simulink model "DY05S600_robot_controller_main_opensource"  (R2020a)
settings: Solver=FixedStepAuto  StartTime=0.0  StopTime=inf  FixedStep=SAMPLE_TIME  RelTol=1e-3
(part 2 of 2)

== matlab function DY05S600_robot_controller_main_opensource/ATS_controller/fuzzy_membership_function12 ==
  data: x input; beta output; wdot output
function [beta,wdot] = fcn(x)

%xm是规则中心
xm=zeros(5,4);
for j=1:5
    xm(j,1)=-0.26+0.13*(j-1)+0.1;
end
for j=6:10
    xm(j-5,2)=-0.18+0.09*(j-5-1)+0.1;
end
for j=11:15
    xm(j-10,3)=-0.14+0.07*(j-10-1)+0.1;
end
for j=16:20
    xm(j-15,4)=-0.4+0.2*(j-15-1)+0.1;
end



%xm是规则中心从小值到大值排列,x是前件变量,
r=length(xm(:,1)); %length(xm)是规则数量r
n=length(xm(1,:));%length(x)是前件变量维度
%初始化隶属度函数
ux=zeros(r,n);

for k=1:n
    if x(k)<=xm(1,k)   %论域左边界外
        ux(1,k)=1;
    end
    if x(k)>=xm(r,k)   %论域右边界外
        ux(r,k)=1;
    end
    for i=1:r-1  %从左到右只计算下降的隶属度函数
        if x(k)>=xm(i,k)&&x(k)<=xm(i+1,k)
           ux(i,k)=0.5*sin(pi*(x(k)-xm(i,k))/abs(xm(i,k)-xm(i+1,k))+0.5*pi)+0.5; %一种具有一阶可导性的四边形家族隶属度函数
        end
    end
    for i=2:r  %从左到右只计算上升的隶属度函数
        if x(k)>=xm(i-1,k)&&x(k)<=xm(i,k)
           ux(i,k)=0.5*sin(pi*(x(k)-xm(i,k))/abs(xm(i-1,k)-xm(i,k))+0.5*pi)+0.5;
        end
    end
end

kx=1;
jz=1;
[beta,wdot]= fuzzyoutput(ux,x,xm,kx,jz);

% function  [Basic,beta]= sumfuzzy_test(x) 
% ux=x;
% im=1;
% jm=0;
% bias=1;
% Basic=0;
% dem=length(ux(:,1))^length(ux(1,:)); %隶属度函数的重数数量
% beta=zeros(dem,1);
% [Basic,beta] = myfun(im,jm,ux,bias,Basic,beta);
% function [Basic,beta,jm] = myfun(im,jm,ux,bias,Basic,beta) 
% %针对ux隶属度函数矩阵的中心平均解模糊，初值赋为1,0，ux，1，0，执行的是多重求和
%     if  im > length(ux(1,:))    %length(ux(1,:))为前件输入的维度
%         Basic = Basic + bias;
%         jm=jm+1;                %相对于i1...in规则编号，此处是从最后一列填满到第一列（i1,...,in）
%         beta(jm,1)=bias;        %beta(i1,...,in)*xk*z(i6,j)
%     else
%         for km=1:length(ux(:,1))   %length(ux(:,1))为规则数量
%             bias_last = bias;
%             bias = bias* ux(km,im);
%             im = im+1;
%             [Basic,beta,jm] = myfun(im,jm,ux,bias,Basic,beta); %递归，拦在这里一直到function执行结束,每执行一次就会多一个for循环（每次跳出就是再一次的for内循环）
%             im = im-1; 
%             bias  = bias_last;
%         end
%     end
% end


end

== matlab function DY05S600_robot_controller_main_opensource/ATS_controller/fuzzy_membership_function9 ==
  data: x input; beta output; wdot output
function [beta,wdot] = fcn(x)

%xm是规则中心
xm=zeros(5,4);
for j=1:5
    xm(j,1)=-0.26+0.13*(j-1)+0.1;
end
for j=6:10
    xm(j-5,2)=-0.18+0.09*(j-5-1)+0.1;
end
for j=11:15
    xm(j-10,3)=-0.14+0.07*(j-10-1)+0.1;
end
for j=16:20
    xm(j-15,4)=-0.4+0.2*(j-15-1)+0.1;
end



%xm是规则中心从小值到大值排列,x是前件变量,
r=length(xm(:,1)); %length(xm)是规则数量r
n=length(xm(1,:));%length(x)是前件变量维度
%初始化隶属度函数
ux=zeros(r,n);

for k=1:n
    if x(k)<=xm(1,k)   %论域左边界外
        ux(1,k)=1;
    end
    if x(k)>=xm(r,k)   %论域右边界外
        ux(r,k)=1;
    end
    for i=1:r-1  %从左到右只计算下降的隶属度函数
        if x(k)>=xm(i,k)&&x(k)<=xm(i+1,k)
           ux(i,k)=0.5*sin(pi*(x(k)-xm(i,k))/abs(xm(i,k)-xm(i+1,k))+0.5*pi)+0.5; %一种具有一阶可导性的四边形家族隶属度函数
        end
    end
    for i=2:r  %从左到右只计算上升的隶属度函数
        if x(k)>=xm(i-1,k)&&x(k)<=xm(i,k)
           ux(i,k)=0.5*sin(pi*(x(k)-xm(i,k))/abs(xm(i-1,k)-xm(i,k))+0.5*pi)+0.5;
        end
    end
end

kx=1;
jz=1;
[beta,wdot]= fuzzyoutput(ux,x,xm,kx,jz);

% function  [Basic,beta]= sumfuzzy_test(x) 
% ux=x;
% im=1;
% jm=0;
% bias=1;
% Basic=0;
% dem=length(ux(:,1))^length(ux(1,:)); %隶属度函数的重数数量
% beta=zeros(dem,1);
% [Basic,beta] = myfun(im,jm,ux,bias,Basic,beta);
% function [Basic,beta,jm] = myfun(im,jm,ux,bias,Basic,beta) 
% %针对ux隶属度函数矩阵的中心平均解模糊，初值赋为1,0，ux，1，0，执行的是多重求和
%     if  im > length(ux(1,:))    %length(ux(1,:))为前件输入的维度
%         Basic = Basic + bias;
%         jm=jm+1;                %相对于i1...in规则编号，此处是从最后一列填满到第一列（i1,...,in）
%         beta(jm,1)=bias;        %beta(i1,...,in)*xk*z(i6,j)
%     else
%         for km=1:length(ux(:,1))   %length(ux(:,1))为规则数量
%             bias_last = bias;
%             bias = bias* ux(km,im);
%             im = im+1;
%             [Basic,beta,jm] = myfun(im,jm,ux,bias,Basic,beta); %递归，拦在这里一直到function执行结束,每执行一次就会多一个for循环（每次跳出就是再一次的for内循环）
%             im = im-1; 
%             bias  = bias_last;
%         end
%     end
% end


end

== matlab function DY05S600_robot_controller_main_opensource/ATS_controller/TSfuzzy_system_output13 ==
  data: beta input; w input; AF11 output
function AF11  = fcn(beta,w)

AF11=0;
for i=1:length(beta)
    AF11=AF11+w(i,1)*beta(i,1);
end

end

== matlab function DY05S600_robot_controller_main_opensource/ATS_controller/TSfuzzy_system_output14 ==
  data: beta input; w input; AF11 output
function AF11  = fcn(beta,w)

AF11=0;
for i=1:length(beta)
    AF11=AF11+w(i,1)*beta(i,1);
end

end

== matlab function DY05S600_robot_controller_main_opensource/ATS_controller/TSfuzzy_system_output15 ==
  data: beta input; w input; AF11 output
function AF11  = fcn(beta,w)

AF11=0;
for i=1:length(beta)
    AF11=AF11+w(i,1)*beta(i,1);
end

end

== matlab function DY05S600_robot_controller_main_opensource/ATS_controller/TSfuzzy_system_output16 ==
  data: beta input; w input; AF11 output
function AF11  = fcn(beta,w)

AF11=0;
for i=1:length(beta)
    AF11=AF11+w(i,1)*beta(i,1);
end

end

== matlab function DY05S600_robot_controller_main_opensource/ATS_controller/controller4 ==
  data: AF11 input; AF12 input; AF21 input; AF22 input; K1 input; K2 input; u1 output; u2 output; x1 input; x2 input; dag output
function [u1,u2,dag]  = fcn(AF11,AF12,AF21,AF22,K1,K2,x1,x2)

b1=0.1;
b2=0.01;

dag=0.8*pi/180;

% u1=-1/b1*((0+AF11)*x1+(0+AF12)*x2+K1*x1/dag^2);
% 
% u2=-1/b2*((0+AF21)*x1+(0+AF22)*x2+K2*x2/dag^2);

% dagx1=0.5*pi/180;
% satx1=0;
% if abs(x1)<dagx1
%     satx1=sign(x1);
% else
%     satx1=x1/dagx1;
% end

   
u1=-1/b1*((0.3+AF11)*x1+(0+AF12)*x2+K1*4/pi*atan(x1/dag));

u2=-1/b2*((2+AF21)*x1+(0.4+AF22)*x2+K2*4/pi*atan(x2/dag));


end

== matlab function DY05S600_robot_controller_main_opensource/ATS_controller/fuzzy_membership_function13 ==
  data: x input; beta output; wdot output
function [beta,wdot] = fcn(x)

%xm是规则中心
xm=zeros(5,4);
for j=1:5
    xm(j,1)=-0.26+0.13*(j-1)+0.1;
end
for j=6:10
    xm(j-5,2)=-0.18+0.09*(j-5-1)+0.1;
end
for j=11:15
    xm(j-10,3)=-0.14+0.07*(j-10-1)+0.1;
end
for j=16:20
    xm(j-15,4)=-0.4+0.2*(j-15-1)+0.1;
end



%xm是规则中心从小值到大值排列,x是前件变量,
r=length(xm(:,1)); %length(xm)是规则数量r
n=length(xm(1,:));%length(x)是前件变量维度
%初始化隶属度函数
ux=zeros(r,n);

for k=1:n
    if x(k)<=xm(1,k)   %论域左边界外
        ux(1,k)=1;
    end
    if x(k)>=xm(r,k)   %论域右边界外
        ux(r,k)=1;
    end
    for i=1:r-1  %从左到右只计算下降的隶属度函数
        if x(k)>=xm(i,k)&&x(k)<=xm(i+1,k)
           ux(i,k)=0.5*sin(pi*(x(k)-xm(i,k))/abs(xm(i,k)-xm(i+1,k))+0.5*pi)+0.5; %一种具有一阶可导性的四边形家族隶属度函数
        end
    end
    for i=2:r  %从左到右只计算上升的隶属度函数
        if x(k)>=xm(i-1,k)&&x(k)<=xm(i,k)
           ux(i,k)=0.5*sin(pi*(x(k)-xm(i,k))/abs(xm(i-1,k)-xm(i,k))+0.5*pi)+0.5;
        end
    end
end

kx=1;
jz=1;
[beta,wdot]= fuzzyoutput(ux,x,xm,kx,jz);

% function  [Basic,beta]= sumfuzzy_test(x) 
% ux=x;
% im=1;
% jm=0;
% bias=1;
% Basic=0;
% dem=length(ux(:,1))^length(ux(1,:)); %隶属度函数的重数数量
% beta=zeros(dem,1);
% [Basic,beta] = myfun(im,jm,ux,bias,Basic,beta);
% function [Basic,beta,jm] = myfun(im,jm,ux,bias,Basic,beta) 
% %针对ux隶属度函数矩阵的中心平均解模糊，初值赋为1,0，ux，1，0，执行的是多重求和
%     if  im > length(ux(1,:))    %length(ux(1,:))为前件输入的维度
%         Basic = Basic + bias;
%         jm=jm+1;                %相对于i1...in规则编号，此处是从最后一列填满到第一列（i1,...,in）
%         beta(jm,1)=bias;        %beta(i1,...,in)*xk*z(i6,j)
%     else
%         for km=1:length(ux(:,1))   %length(ux(:,1))为规则数量
%             bias_last = bias;
%             bias = bias* ux(km,im);
%             im = im+1;
%             [Basic,beta,jm] = myfun(im,jm,ux,bias,Basic,beta); %递归，拦在这里一直到function执行结束,每执行一次就会多一个for循环（每次跳出就是再一次的for内循环）
%             im = im-1; 
%             bias  = bias_last;
%         end
%     end
% end


end

== matlab function DY05S600_robot_controller_main_opensource/ATS_controller/fuzzy_membership_function14 ==
  data: x input; beta output; wdot output
function [beta,wdot] = fcn(x)

%xm是规则中心
xm=zeros(5,4);
for j=1:5
    xm(j,1)=-0.26+0.13*(j-1)+0.1;
end
for j=6:10
    xm(j-5,2)=-0.18+0.09*(j-5-1)+0.1;
end
for j=11:15
    xm(j-10,3)=-0.14+0.07*(j-10-1)+0.1;
end
for j=16:20
    xm(j-15,4)=-0.4+0.2*(j-15-1)+0.1;
end



%xm是规则中心从小值到大值排列,x是前件变量,
r=length(xm(:,1)); %length(xm)是规则数量r
n=length(xm(1,:));%length(x)是前件变量维度
%初始化隶属度函数
ux=zeros(r,n);

for k=1:n
    if x(k)<=xm(1,k)   %论域左边界外
        ux(1,k)=1;
    end
    if x(k)>=xm(r,k)   %论域右边界外
        ux(r,k)=1;
    end
    for i=1:r-1  %从左到右只计算下降的隶属度函数
        if x(k)>=xm(i,k)&&x(k)<=xm(i+1,k)
           ux(i,k)=0.5*sin(pi*(x(k)-xm(i,k))/abs(xm(i,k)-xm(i+1,k))+0.5*pi)+0.5; %一种具有一阶可导性的四边形家族隶属度函数
        end
    end
    for i=2:r  %从左到右只计算上升的隶属度函数
        if x(k)>=xm(i-1,k)&&x(k)<=xm(i,k)
           ux(i,k)=0.5*sin(pi*(x(k)-xm(i,k))/abs(xm(i-1,k)-xm(i,k))+0.5*pi)+0.5;
        end
    end
end

kx=1;
jz=1;
[beta,wdot]= fuzzyoutput(ux,x,xm,kx,jz);

% function  [Basic,beta]= sumfuzzy_test(x) 
% ux=x;
% im=1;
% jm=0;
% bias=1;
% Basic=0;
% dem=length(ux(:,1))^length(ux(1,:)); %隶属度函数的重数数量
% beta=zeros(dem,1);
% [Basic,beta] = myfun(im,jm,ux,bias,Basic,beta);
% function [Basic,beta,jm] = myfun(im,jm,ux,bias,Basic,beta) 
% %针对ux隶属度函数矩阵的中心平均解模糊，初值赋为1,0，ux，1，0，执行的是多重求和
%     if  im > length(ux(1,:))    %length(ux(1,:))为前件输入的维度
%         Basic = Basic + bias;
%         jm=jm+1;                %相对于i1...in规则编号，此处是从最后一列填满到第一列（i1,...,in）
%         beta(jm,1)=bias;        %beta(i1,...,in)*xk*z(i6,j)
%     else
%         for km=1:length(ux(:,1))   %length(ux(:,1))为规则数量
%             bias_last = bias;
%             bias = bias* ux(km,im);
%             im = im+1;
%             [Basic,beta,jm] = myfun(im,jm,ux,bias,Basic,beta); %递归，拦在这里一直到function执行结束,每执行一次就会多一个for循环（每次跳出就是再一次的for内循环）
%             im = im-1; 
%             bias  = bias_last;
%         end
%     end
% end


end

== matlab function DY05S600_robot_controller_main_opensource/ATS_controller/fuzzy_membership_function15 ==
  data: x input; beta output; wdot output
function [beta,wdot] = fcn(x)

%xm是规则中心
xm=zeros(5,4);
for j=1:5
    xm(j,1)=-0.26+0.13*(j-1)+0.1;
end
for j=6:10
    xm(j-5,2)=-0.18+0.09*(j-5-1)+0.1;
end
for j=11:15
    xm(j-10,3)=-0.14+0.07*(j-10-1)+0.1;
end
for j=16:20
    xm(j-15,4)=-0.4+0.2*(j-15-1)+0.1;
end


%xm是规则中心从小值到大值排列,x是前件变量,
r=length(xm(:,1)); %length(xm)是规则数量r
n=length(xm(1,:));%length(x)是前件变量维度
%初始化隶属度函数
ux=zeros(r,n);

for k=1:n
    if x(k)<=xm(1,k)   %论域左边界外
        ux(1,k)=1;
    end
    if x(k)>=xm(r,k)   %论域右边界外
        ux(r,k)=1;
    end
    for i=1:r-1  %从左到右只计算下降的隶属度函数
        if x(k)>=xm(i,k)&&x(k)<=xm(i+1,k)
           ux(i,k)=0.5*sin(pi*(x(k)-xm(i,k))/abs(xm(i,k)-xm(i+1,k))+0.5*pi)+0.5; %一种具有一阶可导性的四边形家族隶属度函数
        end
    end
    for i=2:r  %从左到右只计算上升的隶属度函数
        if x(k)>=xm(i-1,k)&&x(k)<=xm(i,k)
           ux(i,k)=0.5*sin(pi*(x(k)-xm(i,k))/abs(xm(i-1,k)-xm(i,k))+0.5*pi)+0.5;
        end
    end
end

kx=1;
jz=1;
[beta,wdot]= fuzzyoutput(ux,x,xm,kx,jz);

% function  [Basic,beta]= sumfuzzy_test(x) 
% ux=x;
% im=1;
% jm=0;
% bias=1;
% Basic=0;
% dem=length(ux(:,1))^length(ux(1,:)); %隶属度函数的重数数量
% beta=zeros(dem,1);
% [Basic,beta] = myfun(im,jm,ux,bias,Basic,beta);
% function [Basic,beta,jm] = myfun(im,jm,ux,bias,Basic,beta) 
% %针对ux隶属度函数矩阵的中心平均解模糊，初值赋为1,0，ux，1，0，执行的是多重求和
%     if  im > length(ux(1,:))    %length(ux(1,:))为前件输入的维度
%         Basic = Basic + bias;
%         jm=jm+1;                %相对于i1...in规则编号，此处是从最后一列填满到第一列（i1,...,in）
%         beta(jm,1)=bias;        %beta(i1,...,in)*xk*z(i6,j)
%     else
%         for km=1:length(ux(:,1))   %length(ux(:,1))为规则数量
%             bias_last = bias;
%             bias = bias* ux(km,im);
%             im = im+1;
%             [Basic,beta,jm] = myfun(im,jm,ux,bias,Basic,beta); %递归，拦在这里一直到function执行结束,每执行一次就会多一个for循环（每次跳出就是再一次的for内循环）
%             im = im-1; 
%             bias  = bias_last;
%         end
%     end
% end


end

== matlab function DY05S600_robot_controller_main_opensource/ATS_controller/fuzzy_membership_function16 ==
  data: x input; beta output; wdot output
function [beta,wdot] = fcn(x)

%xm是规则中心
xm=zeros(5,4);
for j=1:5
    xm(j,1)=-0.26+0.13*(j-1)+0.1;
end
for j=6:10
    xm(j-5,2)=-0.18+0.09*(j-5-1)+0.1;
end
for j=11:15
    xm(j-10,3)=-0.14+0.07*(j-10-1)+0.1;
end
for j=16:20
    xm(j-15,4)=-0.4+0.2*(j-15-1)+0.1;
end



%xm是规则中心从小值到大值排列,x是前件变量,
r=length(xm(:,1)); %length(xm)是规则数量r
n=length(xm(1,:));%length(x)是前件变量维度
%初始化隶属度函数
ux=zeros(r,n);

for k=1:n
    if x(k)<=xm(1,k)   %论域左边界外
        ux(1,k)=1;
    end
    if x(k)>=xm(r,k)   %论域右边界外
        ux(r,k)=1;
    end
    for i=1:r-1  %从左到右只计算下降的隶属度函数
        if x(k)>=xm(i,k)&&x(k)<=xm(i+1,k)
           ux(i,k)=0.5*sin(pi*(x(k)-xm(i,k))/abs(xm(i,k)-xm(i+1,k))+0.5*pi)+0.5; %一种具有一阶可导性的四边形家族隶属度函数
        end
    end
    for i=2:r  %从左到右只计算上升的隶属度函数
        if x(k)>=xm(i-1,k)&&x(k)<=xm(i,k)
           ux(i,k)=0.5*sin(pi*(x(k)-xm(i,k))/abs(xm(i-1,k)-xm(i,k))+0.5*pi)+0.5;
        end
    end
end

kx=1;
jz=1;
[beta,wdot]= fuzzyoutput(ux,x,xm,kx,jz);

% function  [Basic,beta]= sumfuzzy_test(x) 
% ux=x;
% im=1;
% jm=0;
% bias=1;
% Basic=0;
% dem=length(ux(:,1))^length(ux(1,:)); %隶属度函数的重数数量
% beta=zeros(dem,1);
% [Basic,beta] = myfun(im,jm,ux,bias,Basic,beta);
% function [Basic,beta,jm] = myfun(im,jm,ux,bias,Basic,beta) 
% %针对ux隶属度函数矩阵的中心平均解模糊，初值赋为1,0，ux，1，0，执行的是多重求和
%     if  im > length(ux(1,:))    %length(ux(1,:))为前件输入的维度
%         Basic = Basic + bias;
%         jm=jm+1;                %相对于i1...in规则编号，此处是从最后一列填满到第一列（i1,...,in）
%         beta(jm,1)=bias;        %beta(i1,...,in)*xk*z(i6,j)
%     else
%         for km=1:length(ux(:,1))   %length(ux(:,1))为规则数量
%             bias_last = bias;
%             bias = bias* ux(km,im);
%             im = im+1;
%             [Basic,beta,jm] = myfun(im,jm,ux,bias,Basic,beta); %递归，拦在这里一直到function执行结束,每执行一次就会多一个for循环（每次跳出就是再一次的for内循环）
%             im = im-1; 
%             bias  = bias_last;
%         end
%     end
% end


end

== matlab function DY05S600_robot_controller_main_opensource/ATS_controller/K_comp1 ==
  data: k1 input; x1 input; x2 input; y output; k2 input
function y   = fcn(k1,x1,x2,k2)

x=abs(x1*180/pi)-0.01;

ux=zeros(13,1);
%%x1 13条模糊规则
h1=0.2;%%规则间距


if x<=0
    ux(1,1)=1;
end

if x>=0&&x<=0.2
    ux(1,1)=0.5*sin(pi*(x-(0))/h1+0.5*pi)+0.5;
end

if x>=0&&x<=0.4
    ux(2,1)=0.5*sin(pi*(x-(0.2))/h1+0.5*pi)+0.5;
end

if x>=0.2&&x<=0.6
    ux(3,1)=0.5*sin(pi*(x-(0.4))/h1+0.5*pi)+0.5;
end

if x>=0.4&&x<=0.8
    ux(4,1)=0.5*sin(pi*(x-(0.6))/h1+0.5*pi)+0.5;
end

if x>=0.6&&x<=1
    ux(5,1)=0.5*sin(pi*(x-(0.8))/h1+0.5*pi)+0.5;
end

if x>=0.8&&x<=1.2
    ux(6,1)=0.5*sin(pi*(x-(1))/h1+0.5*pi)+0.5;
end

if x>=1&&x<=1.4
    ux(7,1)=0.5*sin(pi*(x-(1.2))/h1+0.5*pi)+0.5;
end

if x>=1.2&&x<=1.6
    ux(8,1)=0.5*sin(pi*(x-(1.4))/h1+0.5*pi)+0.5;
end

if x>=1.4&&x<=1.8
    ux(9,1)=0.5*sin(pi*(x-(1.6))/h1+0.5*pi)+0.5;
end

if x>=1.6&&x<=2
    ux(10,1)=0.5*sin(pi*(x-(1.8))/h1+0.5*pi)+0.5;
end

if x>=1.8&&x<=2.2
    ux(11,1)=0.5*sin(pi*(x-(2))/h1+0.5*pi)+0.5;
end

if x>=2&&x<=2.4
    ux(12,1)=0.5*sin(pi*(x-(2.2))/h1+0.5*pi)+0.5;
end

if x>=2.2&&x<=2.4
    ux(13,1)=0.5*sin(pi*(x-(2.4))/h1+0.5*pi)+0.5;
end

if x>2.4
    ux(13,1)=1;
end

%中心平均解模糊
Basic=0;
for i=1:13
    Basic=Basic+ux(i,1);
end

beta=zeros(13,1);
for i=1:13
    beta(i,1)=ux(i,1)/Basic;
end

w=[0;1;0.95;0.9;0.85;0.8;0.75;0.7;0.65;0.6;0.55;0.5;0.45/exp(-2.4)*exp(-x)];

f=0;
for i=1:13
    f=f+w(i,1)*beta(i,1);
end

y1=f*k1;
y2=f*k2;
y=[y1,y2]';

end

== matlab function DY05S600_robot_controller_main_opensource/ATS_controller/TSfuzzy_system_output17 ==
  data: beta input; w input; AF11 output
function AF11  = fcn(beta,w)

AF11=0;
for i=1:length(beta)
    AF11=AF11+w(i,1)*beta(i,1);
end

end

== matlab function DY05S600_robot_controller_main_opensource/ATS_controller/TSfuzzy_system_output18 ==
  data: beta input; w input; AF11 output
function AF11  = fcn(beta,w)

AF11=0;
for i=1:length(beta)
    AF11=AF11+w(i,1)*beta(i,1);
end

end

== matlab function DY05S600_robot_controller_main_opensource/ATS_controller/TSfuzzy_system_output19 ==
  data: beta input; w input; AF11 output
function AF11  = fcn(beta,w)

AF11=0;
for i=1:length(beta)
    AF11=AF11+w(i,1)*beta(i,1);
end

end

== matlab function DY05S600_robot_controller_main_opensource/ATS_controller/TSfuzzy_system_output20 ==
  data: beta input; w input; AF11 output
function AF11  = fcn(beta,w)

AF11=0;
for i=1:length(beta)
    AF11=AF11+w(i,1)*beta(i,1);
end

end

== matlab function DY05S600_robot_controller_main_opensource/ATS_controller/controller5 ==
  data: AF11 input; AF12 input; AF21 input; AF22 input; K1 input; K2 input; u1 output; u2 output; x1 input; x2 input; dag output
function [u1,u2,dag]  = fcn(AF11,AF12,AF21,AF22,K1,K2,x1,x2)

b1=0.1;
b2=0.01;

dag=1*pi/180;

% u1=-1/b1*((0+AF11)*x1+(0+AF12)*x2+K1*x1/dag^2);
% 
% u2=-1/b2*((0+AF21)*x1+(0+AF22)*x2+K2*x2/dag^2);

% dagx1=0.5*pi/180;
% satx1=0;
% if abs(x1)<dagx1
%     satx1=sign(x1);
% else
%     satx1=x1/dagx1;
% end

   
u1=-1/b1*((0.1+AF11)*x1+(0+AF12)*x2+K1*4/pi*atan(x1/dag));

u2=-1/b2*((2+AF21)*x1+(0.1+AF22)*x2+K2*4/pi*atan(x2/dag));


end

== matlab function DY05S600_robot_controller_main_opensource/ATS_controller/fuzzy_membership_function17 ==
  data: x input; beta output; wdot output
function [beta,wdot] = fcn(x)

%xm是规则中心
xm=zeros(5,4);
for j=1:5
    xm(j,1)=-0.26+0.13*(j-1)+0.1;
end
for j=6:10
    xm(j-5,2)=-0.18+0.09*(j-5-1)+0.1;
end
for j=11:15
    xm(j-10,3)=-0.14+0.07*(j-10-1)+0.1;
end
for j=16:20
    xm(j-15,4)=-0.4+0.2*(j-15-1)+0.1;
end



%xm是规则中心从小值到大值排列,x是前件变量,
r=length(xm(:,1)); %length(xm)是规则数量r
n=length(xm(1,:));%length(x)是前件变量维度
%初始化隶属度函数
ux=zeros(r,n);

for k=1:n
    if x(k)<=xm(1,k)   %论域左边界外
        ux(1,k)=1;
    end
    if x(k)>=xm(r,k)   %论域右边界外
        ux(r,k)=1;
    end
    for i=1:r-1  %从左到右只计算下降的隶属度函数
        if x(k)>=xm(i,k)&&x(k)<=xm(i+1,k)
           ux(i,k)=0.5*sin(pi*(x(k)-xm(i,k))/abs(xm(i,k)-xm(i+1,k))+0.5*pi)+0.5; %一种具有一阶可导性的四边形家族隶属度函数
        end
    end
    for i=2:r  %从左到右只计算上升的隶属度函数
        if x(k)>=xm(i-1,k)&&x(k)<=xm(i,k)
           ux(i,k)=0.5*sin(pi*(x(k)-xm(i,k))/abs(xm(i-1,k)-xm(i,k))+0.5*pi)+0.5;
        end
    end
end

kx=1;
jz=1;
[beta,wdot]= fuzzyoutput(ux,x,xm,kx,jz);

% function  [Basic,beta]= sumfuzzy_test(x) 
% ux=x;
% im=1;
% jm=0;
% bias=1;
% Basic=0;
% dem=length(ux(:,1))^length(ux(1,:)); %隶属度函数的重数数量
% beta=zeros(dem,1);
% [Basic,beta] = myfun(im,jm,ux,bias,Basic,beta);
% function [Basic,beta,jm] = myfun(im,jm,ux,bias,Basic,beta) 
% %针对ux隶属度函数矩阵的中心平均解模糊，初值赋为1,0，ux，1，0，执行的是多重求和
%     if  im > length(ux(1,:))    %length(ux(1,:))为前件输入的维度
%         Basic = Basic + bias;
%         jm=jm+1;                %相对于i1...in规则编号，此处是从最后一列填满到第一列（i1,...,in）
%         beta(jm,1)=bias;        %beta(i1,...,in)*xk*z(i6,j)
%     else
%         for km=1:length(ux(:,1))   %length(ux(:,1))为规则数量
%             bias_last = bias;
%             bias = bias* ux(km,im);
%             im = im+1;
%             [Basic,beta,jm] = myfun(im,jm,ux,bias,Basic,beta); %递归，拦在这里一直到function执行结束,每执行一次就会多一个for循环（每次跳出就是再一次的for内循环）
%             im = im-1; 
%             bias  = bias_last;
%         end
%     end
% end


end

== matlab function DY05S600_robot_controller_main_opensource/ATS_controller/fuzzy_membership_function18 ==
  data: x input; beta output; wdot output
function [beta,wdot] = fcn(x)

%xm是规则中心
xm=zeros(5,4);
for j=1:5
    xm(j,1)=-0.26+0.13*(j-1)+0.1;
end
for j=6:10
    xm(j-5,2)=-0.18+0.09*(j-5-1)+0.1;
end
for j=11:15
    xm(j-10,3)=-0.14+0.07*(j-10-1)+0.1;
end
for j=16:20
    xm(j-15,4)=-0.4+0.2*(j-15-1)+0.1;
end



%xm是规则中心从小值到大值排列,x是前件变量,
r=length(xm(:,1)); %length(xm)是规则数量r
n=length(xm(1,:));%length(x)是前件变量维度
%初始化隶属度函数
ux=zeros(r,n);

for k=1:n
    if x(k)<=xm(1,k)   %论域左边界外
        ux(1,k)=1;
    end
    if x(k)>=xm(r,k)   %论域右边界外
        ux(r,k)=1;
    end
    for i=1:r-1  %从左到右只计算下降的隶属度函数
        if x(k)>=xm(i,k)&&x(k)<=xm(i+1,k)
           ux(i,k)=0.5*sin(pi*(x(k)-xm(i,k))/abs(xm(i,k)-xm(i+1,k))+0.5*pi)+0.5; %一种具有一阶可导性的四边形家族隶属度函数
        end
    end
    for i=2:r  %从左到右只计算上升的隶属度函数
        if x(k)>=xm(i-1,k)&&x(k)<=xm(i,k)
           ux(i,k)=0.5*sin(pi*(x(k)-xm(i,k))/abs(xm(i-1,k)-xm(i,k))+0.5*pi)+0.5;
        end
    end
end

kx=1;
jz=1;
[beta,wdot]= fuzzyoutput(ux,x,xm,kx,jz);

% function  [Basic,beta]= sumfuzzy_test(x) 
% ux=x;
% im=1;
% jm=0;
% bias=1;
% Basic=0;
% dem=length(ux(:,1))^length(ux(1,:)); %隶属度函数的重数数量
% beta=zeros(dem,1);
% [Basic,beta] = myfun(im,jm,ux,bias,Basic,beta);
% function [Basic,beta,jm] = myfun(im,jm,ux,bias,Basic,beta) 
% %针对ux隶属度函数矩阵的中心平均解模糊，初值赋为1,0，ux，1，0，执行的是多重求和
%     if  im > length(ux(1,:))    %length(ux(1,:))为前件输入的维度
%         Basic = Basic + bias;
%         jm=jm+1;                %相对于i1...in规则编号，此处是从最后一列填满到第一列（i1,...,in）
%         beta(jm,1)=bias;        %beta(i1,...,in)*xk*z(i6,j)
%     else
%         for km=1:length(ux(:,1))   %length(ux(:,1))为规则数量
%             bias_last = bias;
%             bias = bias* ux(km,im);
%             im = im+1;
%             [Basic,beta,jm] = myfun(im,jm,ux,bias,Basic,beta); %递归，拦在这里一直到function执行结束,每执行一次就会多一个for循环（每次跳出就是再一次的for内循环）
%             im = im-1; 
%             bias  = bias_last;
%         end
%     end
% end


end

== matlab function DY05S600_robot_controller_main_opensource/ATS_controller/fuzzy_membership_function19 ==
  data: x input; beta output; wdot output
function [beta,wdot] = fcn(x)

%xm是规则中心
xm=zeros(5,4);
for j=1:5
    xm(j,1)=-0.26+0.13*(j-1)+0.1;
end
for j=6:10
    xm(j-5,2)=-0.18+0.09*(j-5-1)+0.1;
end
for j=11:15
    xm(j-10,3)=-0.14+0.07*(j-10-1)+0.1;
end
for j=16:20
    xm(j-15,4)=-0.4+0.2*(j-15-1)+0.1;
end


%xm是规则中心从小值到大值排列,x是前件变量,
r=length(xm(:,1)); %length(xm)是规则数量r
n=length(xm(1,:));%length(x)是前件变量维度
%初始化隶属度函数
ux=zeros(r,n);

for k=1:n
    if x(k)<=xm(1,k)   %论域左边界外
        ux(1,k)=1;
    end
    if x(k)>=xm(r,k)   %论域右边界外
        ux(r,k)=1;
    end
    for i=1:r-1  %从左到右只计算下降的隶属度函数
        if x(k)>=xm(i,k)&&x(k)<=xm(i+1,k)
           ux(i,k)=0.5*sin(pi*(x(k)-xm(i,k))/abs(xm(i,k)-xm(i+1,k))+0.5*pi)+0.5; %一种具有一阶可导性的四边形家族隶属度函数
        end
    end
    for i=2:r  %从左到右只计算上升的隶属度函数
        if x(k)>=xm(i-1,k)&&x(k)<=xm(i,k)
           ux(i,k)=0.5*sin(pi*(x(k)-xm(i,k))/abs(xm(i-1,k)-xm(i,k))+0.5*pi)+0.5;
        end
    end
end

kx=1;
jz=1;
[beta,wdot]= fuzzyoutput(ux,x,xm,kx,jz);

% function  [Basic,beta]= sumfuzzy_test(x) 
% ux=x;
% im=1;
% jm=0;
% bias=1;
% Basic=0;
% dem=length(ux(:,1))^length(ux(1,:)); %隶属度函数的重数数量
% beta=zeros(dem,1);
% [Basic,beta] = myfun(im,jm,ux,bias,Basic,beta);
% function [Basic,beta,jm] = myfun(im,jm,ux,bias,Basic,beta) 
% %针对ux隶属度函数矩阵的中心平均解模糊，初值赋为1,0，ux，1，0，执行的是多重求和
%     if  im > length(ux(1,:))    %length(ux(1,:))为前件输入的维度
%         Basic = Basic + bias;
%         jm=jm+1;                %相对于i1...in规则编号，此处是从最后一列填满到第一列（i1,...,in）
%         beta(jm,1)=bias;        %beta(i1,...,in)*xk*z(i6,j)
%     else
%         for km=1:length(ux(:,1))   %length(ux(:,1))为规则数量
%             bias_last = bias;
%             bias = bias* ux(km,im);
%             im = im+1;
%             [Basic,beta,jm] = myfun(im,jm,ux,bias,Basic,beta); %递归，拦在这里一直到function执行结束,每执行一次就会多一个for循环（每次跳出就是再一次的for内循环）
%             im = im-1; 
%             bias  = bias_last;
%         end
%     end
% end


end

== matlab function DY05S600_robot_controller_main_opensource/ATS_controller/fuzzy_membership_function20 ==
  data: x input; beta output; wdot output
function [beta,wdot] = fcn(x)

%xm是规则中心
xm=zeros(5,4);
for j=1:5
    xm(j,1)=-0.26+0.13*(j-1)+0.1;
end
for j=6:10
    xm(j-5,2)=-0.18+0.09*(j-5-1)+0.1;
end
for j=11:15
    xm(j-10,3)=-0.14+0.07*(j-10-1)+0.1;
end
for j=16:20
    xm(j-15,4)=-0.4+0.2*(j-15-1)+0.1;
end



%xm是规则中心从小值到大值排列,x是前件变量,
r=length(xm(:,1)); %length(xm)是规则数量r
n=length(xm(1,:));%length(x)是前件变量维度
%初始化隶属度函数
ux=zeros(r,n);

for k=1:n
    if x(k)<=xm(1,k)   %论域左边界外
        ux(1,k)=1;
    end
    if x(k)>=xm(r,k)   %论域右边界外
        ux(r,k)=1;
    end
    for i=1:r-1  %从左到右只计算下降的隶属度函数
        if x(k)>=xm(i,k)&&x(k)<=xm(i+1,k)
           ux(i,k)=0.5*sin(pi*(x(k)-xm(i,k))/abs(xm(i,k)-xm(i+1,k))+0.5*pi)+0.5; %一种具有一阶可导性的四边形家族隶属度函数
        end
    end
    for i=2:r  %从左到右只计算上升的隶属度函数
        if x(k)>=xm(i-1,k)&&x(k)<=xm(i,k)
           ux(i,k)=0.5*sin(pi*(x(k)-xm(i,k))/abs(xm(i-1,k)-xm(i,k))+0.5*pi)+0.5;
        end
    end
end

kx=1;
jz=1;
[beta,wdot]= fuzzyoutput(ux,x,xm,kx,jz);

% function  [Basic,beta]= sumfuzzy_test(x) 
% ux=x;
% im=1;
% jm=0;
% bias=1;
% Basic=0;
% dem=length(ux(:,1))^length(ux(1,:)); %隶属度函数的重数数量
% beta=zeros(dem,1);
% [Basic,beta] = myfun(im,jm,ux,bias,Basic,beta);
% function [Basic,beta,jm] = myfun(im,jm,ux,bias,Basic,beta) 
% %针对ux隶属度函数矩阵的中心平均解模糊，初值赋为1,0，ux，1，0，执行的是多重求和
%     if  im > length(ux(1,:))    %length(ux(1,:))为前件输入的维度
%         Basic = Basic + bias;
%         jm=jm+1;                %相对于i1...in规则编号，此处是从最后一列填满到第一列（i1,...,in）
%         beta(jm,1)=bias;        %beta(i1,...,in)*xk*z(i6,j)
%     else
%         for km=1:length(ux(:,1))   %length(ux(:,1))为规则数量
%             bias_last = bias;
%             bias = bias* ux(km,im);
%             im = im+1;
%             [Basic,beta,jm] = myfun(im,jm,ux,bias,Basic,beta); %递归，拦在这里一直到function执行结束,每执行一次就会多一个for循环（每次跳出就是再一次的for内循环）
%             im = im-1; 
%             bias  = bias_last;
%         end
%     end
% end


end

== matlab function DY05S600_robot_controller_main_opensource/ATS_controller/TSfuzzy_system_output21 ==
  data: beta input; w input; AF11 output
function AF11  = fcn(beta,w)

AF11=0;
for i=1:length(beta)
    AF11=AF11+w(i,1)*beta(i,1);
end

end

== matlab function DY05S600_robot_controller_main_opensource/ATS_controller/TSfuzzy_system_output22 ==
  data: beta input; w input; AF11 output
function AF11  = fcn(beta,w)

AF11=0;
for i=1:length(beta)
    AF11=AF11+w(i,1)*beta(i,1);
end

end

== matlab function DY05S600_robot_controller_main_opensource/ATS_controller/TSfuzzy_system_output23 ==
  data: beta input; w input; AF11 output
function AF11  = fcn(beta,w)

AF11=0;
for i=1:length(beta)
    AF11=AF11+w(i,1)*beta(i,1);
end

end

== matlab function DY05S600_robot_controller_main_opensource/ATS_controller/TSfuzzy_system_output24 ==
  data: beta input; w input; AF11 output
function AF11  = fcn(beta,w)

AF11=0;
for i=1:length(beta)
    AF11=AF11+w(i,1)*beta(i,1);
end

end

== matlab function DY05S600_robot_controller_main_opensource/ATS_controller/controller6 ==
  data: AF11 input; AF12 input; AF21 input; AF22 input; K1 input; K2 input; u1 output; u2 output; x1 input; x2 input; dag output
function [u1,u2,dag]  = fcn(AF11,AF12,AF21,AF22,K1,K2,x1,x2)

b1=0.1;
b2=0.01;

dag=2.7*pi/180;

% u1=-1/b1*((0+AF11)*x1+(0+AF12)*x2+K1*x1/dag^2);
% 
% u2=-1/b2*((0+AF21)*x1+(0+AF22)*x2+K2*x2/dag^2);

% dagx1=0.5*pi/180;
% satx1=0;
% if abs(x1)<dagx1
%     satx1=sign(x1);
% else
%     satx1=x1/dagx1;
% end

% u1=-1/b1*((0.01+AF11)*x1+(0+AF12)*x2+K1*4/pi*atan(x1/dag));
% 
% 
% u2=-1/b2*((1+AF21)*x1+(0.01+AF22)*x2+K2*4/pi*atan(x2/dag));

u1=-1/b1*((0+0.1*AF11)*x1+(0+0.1*AF12)*x2+K1*4/pi*atan(x1/dag));


u2=-1/b2*((0.1+0.1*AF21)*x1+(0+0.1*AF22)*x2+K2*4/pi*atan(x2/dag));

end

== matlab function DY05S600_robot_controller_main_opensource/ATS_controller/fuzzy_membership_function21 ==
  data: x input; beta output; wdot output
function [beta,wdot] = fcn(x)

%xm是规则中心
xm=zeros(5,4);
for j=1:5
    xm(j,1)=-0.26+0.13*(j-1)+0.1;
end
for j=6:10
    xm(j-5,2)=-0.18+0.09*(j-5-1)+0.1;
end
for j=11:15
    xm(j-10,3)=-0.14+0.07*(j-10-1)+0.1;
end
for j=16:20
    xm(j-15,4)=-0.4+0.2*(j-15-1)+0.1;
end



%xm是规则中心从小值到大值排列,x是前件变量,
r=length(xm(:,1)); %length(xm)是规则数量r
n=length(xm(1,:));%length(x)是前件变量维度
%初始化隶属度函数
ux=zeros(r,n);

for k=1:n
    if x(k)<=xm(1,k)   %论域左边界外
        ux(1,k)=1;
    end
    if x(k)>=xm(r,k)   %论域右边界外
        ux(r,k)=1;
    end
    for i=1:r-1  %从左到右只计算下降的隶属度函数
        if x(k)>=xm(i,k)&&x(k)<=xm(i+1,k)
           ux(i,k)=0.5*sin(pi*(x(k)-xm(i,k))/abs(xm(i,k)-xm(i+1,k))+0.5*pi)+0.5; %一种具有一阶可导性的四边形家族隶属度函数
        end
    end
    for i=2:r  %从左到右只计算上升的隶属度函数
        if x(k)>=xm(i-1,k)&&x(k)<=xm(i,k)
           ux(i,k)=0.5*sin(pi*(x(k)-xm(i,k))/abs(xm(i-1,k)-xm(i,k))+0.5*pi)+0.5;
        end
    end
end

kx=1;
jz=1;
[beta,wdot]= fuzzyoutput(ux,x,xm,kx,jz);

% function  [Basic,beta]= sumfuzzy_test(x) 
% ux=x;
% im=1;
% jm=0;
% bias=1;
% Basic=0;
% dem=length(ux(:,1))^length(ux(1,:)); %隶属度函数的重数数量
% beta=zeros(dem,1);
% [Basic,beta] = myfun(im,jm,ux,bias,Basic,beta);
% function [Basic,beta,jm] = myfun(im,jm,ux,bias,Basic,beta) 
% %针对ux隶属度函数矩阵的中心平均解模糊，初值赋为1,0，ux，1，0，执行的是多重求和
%     if  im > length(ux(1,:))    %length(ux(1,:))为前件输入的维度
%         Basic = Basic + bias;
%         jm=jm+1;                %相对于i1...in规则编号，此处是从最后一列填满到第一列（i1,...,in）
%         beta(jm,1)=bias;        %beta(i1,...,in)*xk*z(i6,j)
%     else
%         for km=1:length(ux(:,1))   %length(ux(:,1))为规则数量
%             bias_last = bias;
%             bias = bias* ux(km,im);
%             im = im+1;
%             [Basic,beta,jm] = myfun(im,jm,ux,bias,Basic,beta); %递归，拦在这里一直到function执行结束,每执行一次就会多一个for循环（每次跳出就是再一次的for内循环）
%             im = im-1; 
%             bias  = bias_last;
%         end
%     end
% end


end
